simulink model "Copy_2_of_CDPR"  (R2023b)
settings: Solver=FixedStepAuto  StartTime=0.0  StopTime=10  FixedStep=0.001  RelTol=1e-3
values from neighbouring files (symbols this model uses):
  qi = R\l0    [Initialisation.m]
  R = (sqrt(0.08^2 + 0.005^2/(2*pi))/25)    [DynModel_q.m]    (also in Initialisation.m = (sqrt(0.08^2 + 0.005^2/(2*pi))/25)   * eye(8); Rot.m = Rz * Ry * Rx; Rz.m = [cos(theta) -sin(theta) 0)
  tau_ci = quadprog(H, f, [], [], Aeq, beq, 50*ones(8,1), 5000*ones(8,1))    [Initialisation.m]    (also in TDA.m = u(13:20))
  Xi = [0, 0.0, 1.5, 0, 0, 0]'    [Initialisation.m]
settings Model: Creator=abellila  LastModifiedBy=abellila
settings SolverCC: NumberNewtonIterations=5

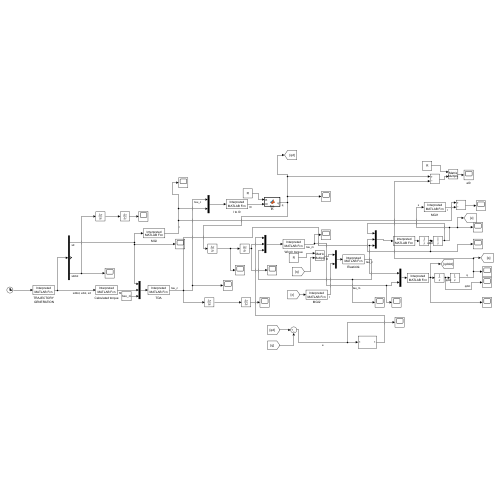
[thumbnail: Simulink's stored preview of the top-level diagram]
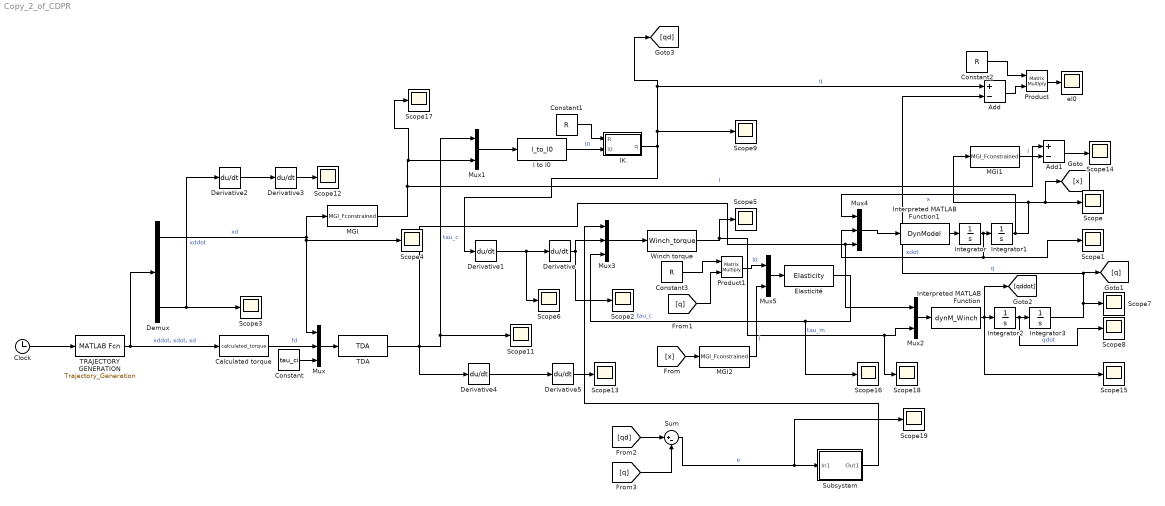
== system Copy_2_of_CDPR ==
  Add : Sum  Inputs=+-
  Add1 : Sum  Inputs=+-
  Calculated torque : MATLABFcn  MATLABFcn=calculated_torque  Output1D=off
  Clock : Clock
  Constant : Constant  Value=tau_ci
  Constant1 : Constant  Value=R
  Constant2 : Constant  Value=R
  Constant3 : Constant  Value=R
  Demux : Demux  Outputs=3
  Derivative{,1..5} (6 alike) : Derivative
  Elasticité : MATLABFcn  MATLABFcn=Elasticity  OutputDimensions=8  OutputSignalType=real  Output1D=off
  IK : MATLAB Function  TreatAsAtomicUnit=on
  Integrator : Integrator  InitialCondition=zeros(6,1)
  Integrator1 : Integrator  InitialCondition=Xi
  Integrator2 : Integrator  InitialCondition=zeros(8,1)
  Integrator3 : Integrator  InitialCondition=qi
  Interpreted MATLAB Function : MATLABFcn  MATLABFcn=dynM_Winch  OutputDimensions=8  Output1D=off
  Interpreted MATLAB Function1 : MATLABFcn  MATLABFcn=DynModel  Output1D=off
  MGI : MATLABFcn  MATLABFcn=MGI_Fconstrained
  MGI1 : MATLABFcn  MATLABFcn=MGI_Fconstrained
  MGI2 : MATLABFcn  MATLABFcn=MGI_Fconstrained
  Mux : Mux  Inputs=3
  Mux1 : Mux  Inputs=2
  Mux2 : Mux  Inputs=2
  Mux3 : Mux  Inputs=3
  Mux4 : Mux  Inputs=3
  Mux5 : Mux  Inputs=2
  Product : Product  Multiplication=Matrix(*)
  Product1 : Product  Multiplication=Matrix(*)
  Scope{,1..9,11..19} (19 alike) : Scope
  Subsystem : Subsystem
  Sum : Sum  Inputs=|+-
  TDA : MATLABFcn  MATLABFcn=TDA  OutputDimensions=8  Output1D=off
  TRAJECTORY GENERATION : MATLABFcn  MATLABFcn=Trajectory_Generation  Output1D=off
  Winch torque : MATLABFcn  MATLABFcn=Winch_torque  OutputDimensions=8  OutputSignalType=real  Output1D=off
  el0 : Scope
  l to l0 : MATLABFcn  MATLABFcn=l_to_l0  OutputDimensions=8  OutputSignalType=real  Output1D=off
  wires:
  Derivative4/1 -> Derivative5/1
  Derivative5/1 -> Scope13/1
  Derivative1/1 -> Derivative/1, Scope6/1
  Derivative2/1 -> Derivative3/1
  Clock/1 -> TRAJECTORY GENERATION/1
  Integrator2/1 -> Scope8/1, Integrator3/1  "qdot"
  Constant1/1 -> IK/1(R)
  Mux/1 -> TDA/1
  Demux/1 -> Mux/1, Scope4/1, MGI/1  "xd"
  Integrator/1 -> Mux4/2, Scope1/1, Integrator1/1  "xdot"
  Constant2/1 -> Product/1
  Add/1 -> Product/2
  Mux3/1 -> Winch torque/1
  Winch torque/1 -> Scope18/1, Mux2/2, Scope5/1  "tau_m"
  Add1/1 -> Scope14/1
  IK/1(q) -> Derivative1/1, [qd], Add/1, Scope9/1  "q"
  TDA/1 -> Derivative4/1, Mux2/1, Mux4/3, Mux1/1, Scope11/1  "tau_c"
  TRAJECTORY GENERATION/1 -> Calculated torque/1, Demux/1  "xddot, xdot, xd"
  Demux/3 -> Derivative2/1, Scope3/1  "xddot"
  Constant/1 -> Mux/3
  Integrator3/1 -> [q], Add/2, Scope7/1  "q"
  Derivative3/1 -> Scope12/1
  Mux2/1 -> Interpreted MATLAB Function/1
  Product/1 -> el0/1
  MGI1/1 -> Add1/2  "l"
  Interpreted MATLAB Function/1 -> Scope15/1, Integrator2/1, [qddot]
  MGI/1 -> Add1/1, Scope17/1, Mux1/2  "l"
  Calculated torque/1 -> Mux/2  "fd"
  l to l0/1 -> IK/2(l0)  "l0"
  Integrator1/1 -> Mux4/1, MGI1/1, [x], Scope/1  "x"
  Mux1/1 -> l to l0/1
  Interpreted MATLAB Function1/1 -> Integrator/1
  Mux4/1 -> Interpreted MATLAB Function1/1
  Mux5/1 -> Elasticité/1
  Derivative/1 -> Scope2/1, Mux3/2
  Constant3/1 -> Product1/1
  Product1/1 -> Mux5/1  "l0"
  [q] -> Product1/2
  [x] -> MGI2/1
  MGI2/1 -> Mux5/2  "l"
  Elasticité/1 -> Scope16/1, Mux3/3  "tau_c"
  Sum/1 -> Scope19/1, Subsystem/1(In1)  "e"
  Subsystem/1(Out1) -> Mux3/1
  [qd] -> Sum/1
  [q] -> Sum/2

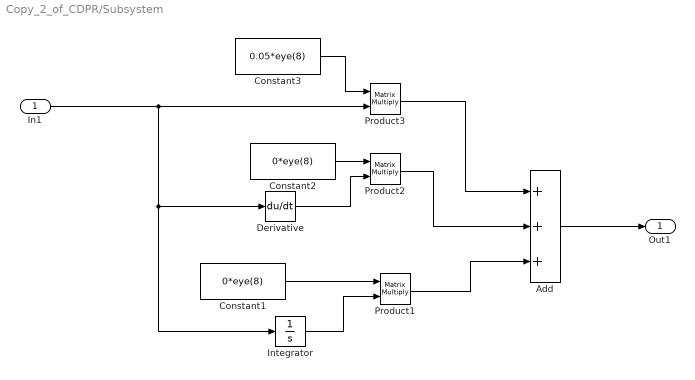
== system Copy_2_of_CDPR/Subsystem ==
  In1 : Inport
  Add : Sum  Inputs=+++
  Constant1 : Constant  Value=0*eye(8)
  Constant2 : Constant  Value=0*eye(8)
  Constant3 : Constant  Value=0.05*eye(8)
  Derivative : Derivative
  Integrator : Integrator
  Product1 : Product  Multiplication=Matrix(*)
  Product2 : Product  Multiplication=Matrix(*)
  Product3 : Product  Multiplication=Matrix(*)
  Out1 : Outport
  wires:
  In1/1 -> Product3/2, Integrator/1, Derivative/1
  Constant2/1 -> Product2/1
  Constant3/1 -> Product3/1
  Derivative/1 -> Product2/2
  Constant1/1 -> Product1/1
  Integrator/1 -> Product1/2
  Add/1 -> Out1/1
  Product3/1 -> Add/1
  Product2/1 -> Add/2
  Product1/1 -> Add/3

== matlab function Copy_2_of_CDPR/IK ==
  data: R input; q output; l0 input
function q = fcn(R, l0)

q = R\l0;
    for i = 1:8
        truncateSignalq(q(i));
    end
